simulink model "pc_audio_sender_v1"  (R2020b)
settings: Solver=VariableStepAuto  StartTime=0.0  StopTime=inf  RelTol=1e-3
undefined symbols (not defined in the file): samples, serial
libraries: instrumentlib x3, simulink x1
settings Model: Creator=adria  LastModifiedBy=tyler

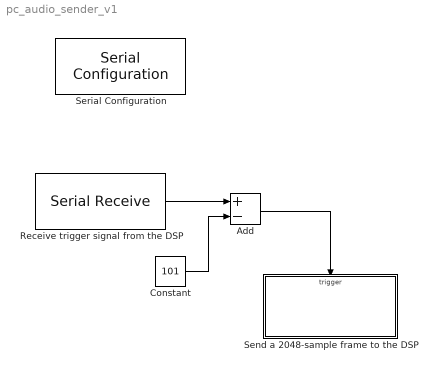
== system pc_audio_sender_v1 ==
  Add : Sum  Inputs=+-
  Constant : Constant  Value=101
  Receive trigger signal from the DSP : instrumentlib/Serial Receive  ComPortMenu=COM6  ComPort=COM6  ObjConstructor=serial('COM6');  Terminator=<none>  DataSize=1  DataType=uint8  EnableBlockingMode=on  ActionDataUnavailable=Output last received value  CustomValue=0  SampleTime=0.01
  Send a 2048-sample frame to the DSP : Subsystem
  Serial Configuration : instrumentlib/Serial Configuration  Priority=-200000  ComPortMenu=COM6  ComPort=COM6  ObjConstructor=serial('COM6');  BaudRate=1e6  DataBits=8  Parity=none  StopBits=1  FlowControl=none  Timeout=10  ByteOrder=LittleEndian
  wires:
  Receive trigger signal from the DSP/1 -> Add/1
  Constant/1 -> Add/2
  Add/1 -> Send a 2048-sample frame to the DSP/Trigger

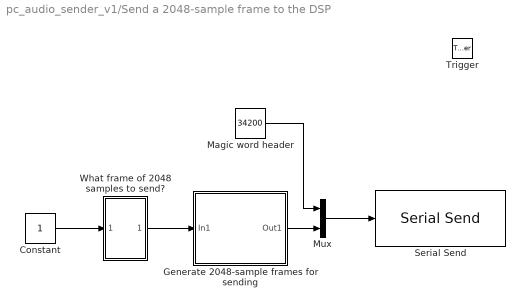
== system pc_audio_sender_v1/Send a 2048-sample frame to the DSP ==
  Trigger : TriggerPort  TriggerType=either  VariantControl=Variant  PortDimensions=1
  Constant : Constant  SampleTime=-1
  Generate 2048-sample frames for sending : Subsystem  TreatAsAtomicUnit=on
  Magic word header : Constant  Value=34200  OutDataTypeStr=uint16  SampleTime=-1
  Mux : Mux  Inputs=2
  Serial Send : instrumentlib/Serial Send  ComPortMenu=COM6  ComPort=COM6  ObjConstructor=serial('COM6');  Terminator=<none>  EnableBlockingMode=on
  What frame of 2048 samples to send? : Subsystem
  wires:
  Mux/1 -> Serial Send/1
  Magic word header/1 -> Mux/1
  Generate 2048-sample frames for sending/1(Out1) -> Mux/2
  Constant/1 -> What frame of 2048 samples to send?/1(In1)
  What frame of 2048 samples to send?/1(Out1) -> Generate 2048-sample frames for sending/1(In1)

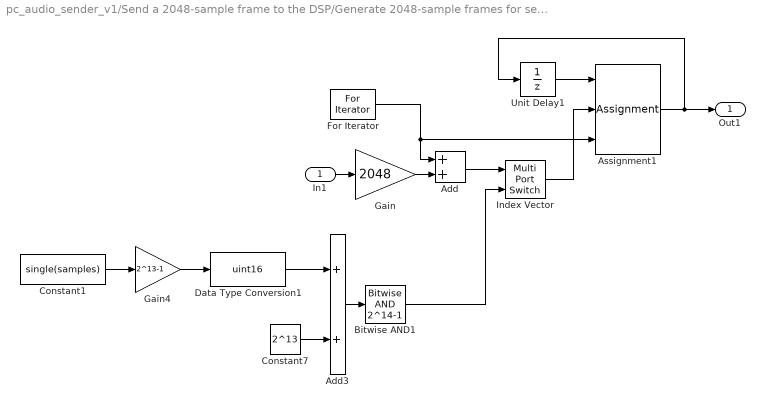
== system pc_audio_sender_v1/Send a 2048-sample frame to the DSP/Generate 2048-sample frames for sending ==
  In1 : Inport
  Add : Sum
  Add3 : Sum
  Assignment1 : Assignment  DiagnosticForDimensions=Warning  IndexOptions=Index vector (port)  Indices=1  OutputSizes=1
  Bitwise AND1 : simulink/Logic and Bit Operations/Bitwise Operator  logicop=AND  UseBitMask=on  BitMask=2^14-1  BitMaskRealWorld=Stored Integer
  Constant1 : Constant  Value=single(samples)  OutDataTypeStr=single
  Constant7 : Constant  Value=2^13  OutDataTypeStr=uint16
  Data Type Conversion1 : DataTypeConversion  OutDataTypeStr=uint16
  For Iterator : ForIterator  ResetStates=reset  IterationLimit=2048
  Gain : Gain  Gain=2048
  Gain4 : Gain  Gain=2^13-1
  Index Vector : MultiPortSwitch  DataPortOrder=Zero-based contiguous  Inputs=1  zeroidx=on
  Unit Delay1 : UnitDelay  InitialCondition=zeros(1,2048)  SampleTime=-1  HasFrameUpgradeWarning=on
  Out1 : Outport
  wires:
  In1/1 -> Gain/1
  Gain/1 -> Add/2
  For Iterator/1 -> Assignment1/3, Add/1
  Add/1 -> Index Vector/1
  Unit Delay1/1 -> Assignment1/1
  Index Vector/1 -> Assignment1/2
  Assignment1/1 -> Unit Delay1/1, Out1/1
  Gain4/1 -> Data Type Conversion1/1
  Constant7/1 -> Add3/2
  Add3/1 -> Bitwise AND1/1
  Data Type Conversion1/1 -> Add3/1
  Constant1/1 -> Gain4/1
  Bitwise AND1/1 -> Index Vector/2

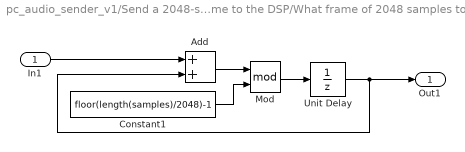
== system pc_audio_sender_v1/Send a 2048-sample frame to the DSP/What frame of 2048 samples to send? ==
  In1 : Inport
  Add : Sum
  Constant1 : Constant  Value=floor(length(samples)/2048)-1
  Mod : Math  Operator=mod  SaturateOnIntegerOverflow=on
  Unit Delay : UnitDelay  SampleTime=-1  HasFrameUpgradeWarning=on
  Out1 : Outport
  wires:
  Unit Delay/1 -> Out1/1, Add/2
  Constant1/1 -> Mod/2
  Add/1 -> Mod/1
  Mod/1 -> Unit Delay/1
  In1/1 -> Add/1
